simulink model "Mathematical_Model"  (R2025a)
settings: Solver=VariableStepAuto  StartTime=0.0  StopTime=10.0  RelTol=1e-3
libraries: simulink x12, slpidlib x4
settings Model: Creator=simon  LastModifiedBy=simon

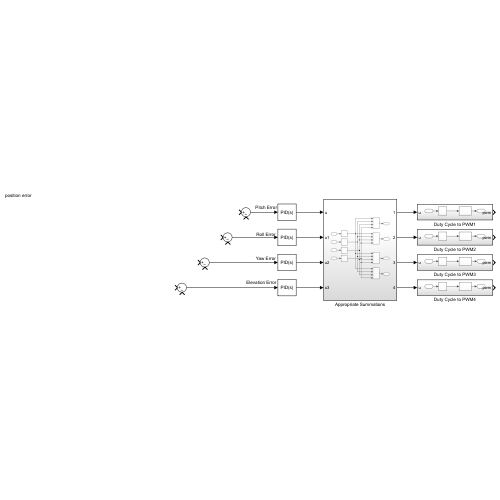
[thumbnail: Simulink's stored preview of the top-level diagram]
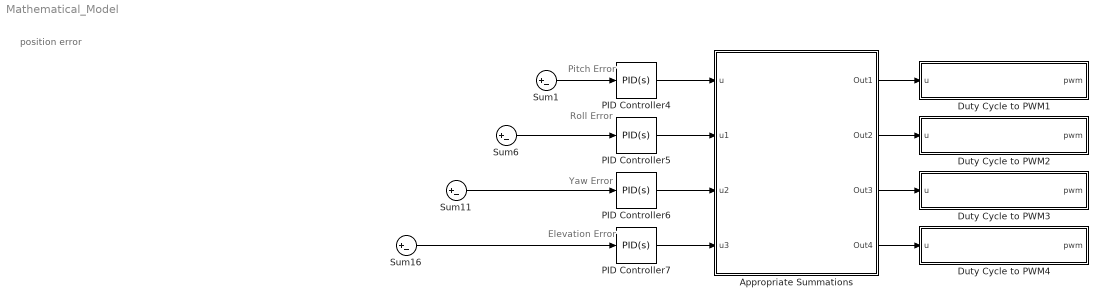
== system Mathematical_Model ==
  note: Pitch Error
  note: Roll Error
  note: Yaw Error
  note: Elevation Error
  note: position error
  Appropriate Summations : Subsystem
  Duty Cycle to PWM1 : Subsystem
  Duty Cycle to PWM2 : Subsystem
  Duty Cycle to PWM3 : Subsystem
  Duty Cycle to PWM4 : Subsystem
  PID Controller{4..7} (4 alike) : slpidlib/PID Controller  Controller=PID  Form=Parallel  TimeDomain=Continuous-time  UseExternalTs=off  SampleTime=-1  IntegratorMethod=Forward Euler  FilterMethod=Forward Euler  ControllerParametersSource=internal  P=1  I=1  UseKiTs=off  D=0  UseExternalDerivativeSource=off  N=100  UseFilter=on  TunerSelectOption=Transfer Function Based (PID Tuner App)  InitialConditionSource=internal  InitialConditionForIntegrator=0  InitialConditionForFilter=0  DifferentiatorICPrevScaledInput=0  ExternalReset=none  TrackingMode=off  Kt=1  LimitOutput=off  SatLimitsSource=internal  UpperSaturationLimit=inf  LowerSaturationLimit=-inf  LinearizeAsGain=on  AntiWindupMode=none  Kb=1  LimitIntegrator=off  UpperIntegratorSaturationLimit=inf  LowerIntegratorSaturationLimit=-inf  POutMin=[]  POutMax=[]  IOutMin=[]  IOutMax=[]  DOutMin=[]  DOutMax=[]  NOutMin=[]  NOutMax=[]  SumOutMin=[]  SumOutMax=[]  SaturationOutMin=[]  SaturationOutMax=[]  PParamMin=[]  PParamMax=[]  IParamMin=[]  IParamMax=[]  DParamMin=[]  DParamMax=[]  NParamMin=[]  NParamMax=[]  KbParamMin=[]  KbParamMax=[]  KtParamMin=[]  KtParamMax=[]  KbOutMin=[]  KbOutMax=[]  KtOutMin=[]  KtOutMax=[]  IntegratorOutMin=[]  IntegratorOutMax=[]  FilterOutMin=[]  FilterOutMax=[]  SumI1OutMin=[]  SumI1OutMax=[]  SumI2OutMin=[]  SumI2OutMax=[]  SumI3OutMin=[]  SumI3OutMax=[]  SumI4OutMin=[]  SumI4OutMax=[]  SumDOutMin=[]  SumDOutMax=[]  DifferentiatorOutMin=[]  DifferentiatorOutMax=[]  FilterDiffOutCoefMin=[]  FilterDiffOutCoefMax=[]  ReciprocalOutMin=[]  ReciprocalOutMax=[]  SumDenOutMin=[]  SumDenOutMax=[]  SumNumOutMin=[]  SumNumOutMax=[]  DivideOutMin=[]  DivideOutMax=[]  UdiffTsProdOutMin=[]  UdiffTsProdOutMax=[]  NTsProdOutMin=[]  NTsProdOutMax=[]  UintegralTsProdOutMin=[]  UintegralTsProdOutMax=[]  UngainTsProdOutMin=[]  UngainTsProdOutMax=[]  ClampingZeroOutDataTypeStr=Inherit: Inherit via back propagation  ClampingZeroOutMin=[]  ClampingZeroOutMax=[]  FilterDenConstantOutDataTypeStr=Inherit: Inherit via back propagation  FilterDenConstantOutMin=[]  FilterDenConstantOutMax=[]  PCopyOutDataTypeStr=Inherit: Inherit via back propagation  PCopyOutMin=[]  PCopyOutMax=[]  NCopyOutDataTypeStr=Inherit: Inherit via back propagation  NCopyOutMin=[]  NCopyOutMax=[]  IntegratorContinuousStateAttributes=''  IntegratorStateMustResolveToSignalObject=off  IntegratorRTWStateStorageClass=Auto  FilterContinuousStateAttributes=''  FilterStateMustResolveToSignalObject=off  FilterRTWStateStorageClass=Auto  ParallelPVariant=InternalParameters  IdealPVariant=Disabled  IVariant=InternalParameters  DVariant=InternalParameters  IntegratorVariant=Continuous  SatVariant=Disabled  AWVariant=Passthrough  PCopyVariant=Disabled  TRVariant=Disabled  FdbkBlocksVariant=Forward  IdealPFdbkVariant=Disabled  SatFdbkVariant=Disabled  DerivativeFilterVariant=ContFilter  NVariant=InternalParameters  NCopyVariant=Disabled  FilterICVariant=InternalICsFilter  IntegratorICVariant=InternalICs  ExternalResetVariant=Disabled  TRSumVariant=Passthrough  SumFdbkVariant=Disabled  SumVariant=Sum_PID  TsampFilterVariant=InternalTs  TsampNgainVariant=Passthrough  TsampIntegralVariant=Disabled_SignalSpec  ExternalSaturationOutDataTypeStr=Inherit: Same as second input  DerivativeSourceVariant=ErrorSignal  PreIntVariant=InternalPreInt
  Sum{1,6,11,16} (4 alike) : Sum  Inputs=|+-
  wires:
  Sum16/1 -> PID Controller7/1
  Sum11/1 -> PID Controller6/1
  Sum6/1 -> PID Controller5/1
  Sum1/1 -> PID Controller4/1
  PID Controller4/1 -> Appropriate Summations/1(u)
  PID Controller5/1 -> Appropriate Summations/2(u1)
  PID Controller6/1 -> Appropriate Summations/3(u2)
  PID Controller7/1 -> Appropriate Summations/4(u3)
  Appropriate Summations/1(Out1) -> Duty Cycle to PWM1/1(u)
  Appropriate Summations/4(Out4) -> Duty Cycle to PWM4/1(u)
  Appropriate Summations/3(Out3) -> Duty Cycle to PWM3/1(u)
  Appropriate Summations/2(Out2) -> Duty Cycle to PWM2/1(u)

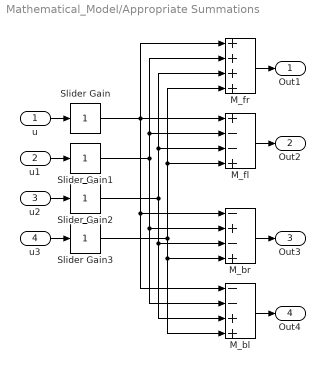
== system Mathematical_Model/Appropriate Summations ==
  u : Inport
  u1 : Inport  Port=2
  u2 : Inport  Port=3
  u3 : Inport  Port=4
  M_bl : Sum  Inputs=--++
  M_br : Sum  Inputs=-+-+
  M_fl : Sum  Inputs=+--+
  M_fr : Sum  Inputs=++++
  Slider Gain{,1..3} (4 alike) : simulink/Math Operations/Slider Gain  gain=1  low=0  high=2
  Out1 : Outport
  Out2 : Outport  Port=2
  Out3 : Outport  Port=3
  Out4 : Outport  Port=4
  wires:
  Slider Gain1/1 -> M_bl/2, M_br/2, M_fl/2, M_fr/2
  Slider Gain3/1 -> M_fl/4, M_fr/4, M_bl/4, M_br/4
  Slider Gain/1 -> M_bl/1, M_br/1, M_fl/1, M_fr/1
  M_bl/1 -> Out4/1
  u/1 -> Slider Gain/1
  M_br/1 -> Out3/1
  u3/1 -> Slider Gain3/1
  Slider Gain2/1 -> M_fl/3, M_fr/3, M_bl/3, M_br/3
  u1/1 -> Slider Gain1/1
  u2/1 -> Slider Gain2/1
  M_fl/1 -> Out2/1
  M_fr/1 -> Out1/1

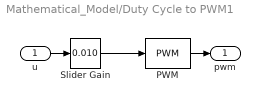
== system Mathematical_Model/Duty Cycle to PWM1 ==
  u : Inport
  PWM : simulink/Discontinuities/PWM  DisableCoverage=on  Period=.1  InitialDelay=0  DisallowZeroDutyCycle=off  RunAtFixedTimeIntervals=off  SampleTime=0.1
  Slider Gain : simulink/Math Operations/Slider Gain  gain=0.010  low=0  high=2
  pwm : Outport
  wires:
  Slider Gain/1 -> PWM/1
  PWM/1 -> pwm/1
  u/1 -> Slider Gain/1

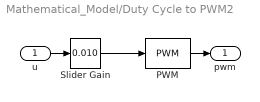
== system Mathematical_Model/Duty Cycle to PWM2 ==
  u : Inport
  PWM : simulink/Discontinuities/PWM  DisableCoverage=on  Period=.1  InitialDelay=0  DisallowZeroDutyCycle=off  RunAtFixedTimeIntervals=off  SampleTime=0.1
  Slider Gain : simulink/Math Operations/Slider Gain  gain=0.010  low=0  high=2
  pwm : Outport
  wires:
  Slider Gain/1 -> PWM/1
  PWM/1 -> pwm/1
  u/1 -> Slider Gain/1

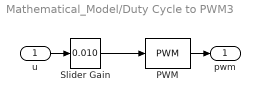
== system Mathematical_Model/Duty Cycle to PWM3 ==
  u : Inport
  PWM : simulink/Discontinuities/PWM  DisableCoverage=on  Period=.1  InitialDelay=0  DisallowZeroDutyCycle=off  RunAtFixedTimeIntervals=off  SampleTime=0.1
  Slider Gain : simulink/Math Operations/Slider Gain  gain=0.010  low=0  high=2
  pwm : Outport
  wires:
  Slider Gain/1 -> PWM/1
  PWM/1 -> pwm/1
  u/1 -> Slider Gain/1

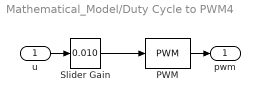
== system Mathematical_Model/Duty Cycle to PWM4 ==
  u : Inport
  PWM : simulink/Discontinuities/PWM  DisableCoverage=on  Period=.1  InitialDelay=0  DisallowZeroDutyCycle=off  RunAtFixedTimeIntervals=off  SampleTime=0.1
  Slider Gain : simulink/Math Operations/Slider Gain  gain=0.010  low=0  high=2
  pwm : Outport
  wires:
  Slider Gain/1 -> PWM/1
  PWM/1 -> pwm/1
  u/1 -> Slider Gain/1
